simulink model "SchemaNL"  (R2020b)
settings: Solver=VariableStepAuto  StartTime=0.0  StopTime=50  RelTol=1e-3
values from neighbouring files (symbols this model uses):
  Kpsi = 0.5    [Coordinate_linearizzazione.m]
  Kx = 0.5    [Coordinate_linearizzazione.m]
  Ky = 0.5    [Coordinate_linearizzazione.m]
undefined symbols (not defined in the file or in its folder): DELTA
settings Model: Creator=teora  LastModifiedBy=teora

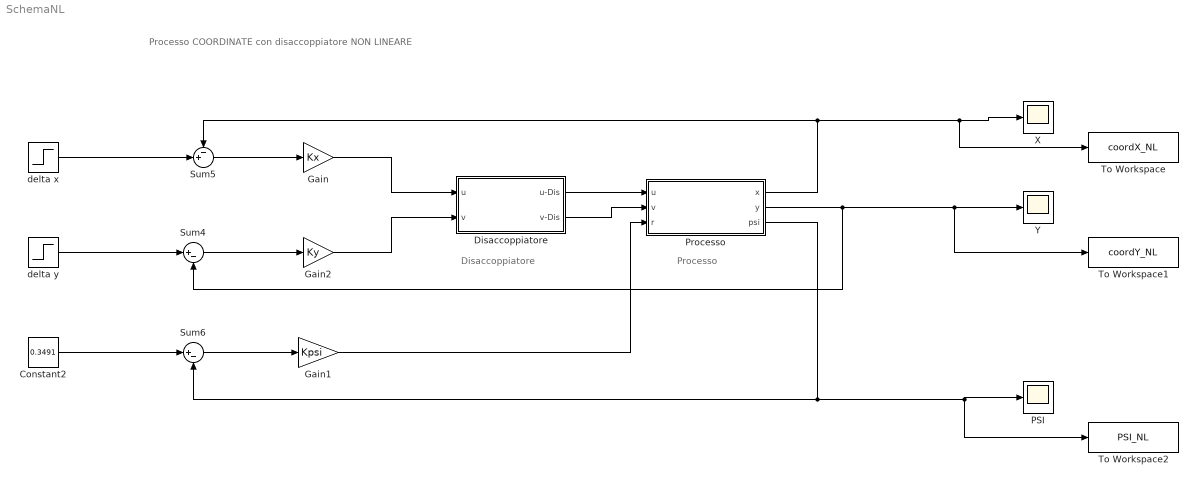
== system SchemaNL ==
  note: Processo
  note: Processo COORDINATE con disaccoppiatore NON LINEARE
  note: Disaccoppiatore
  Constant2 : Constant  Value=0.3491
  Disaccoppiatore : Subsystem
  Gain : Gain  Gain=Kx
  Gain1 : Gain  Gain=Kpsi
  Gain2 : Gain  Gain=Ky
  PSI : Scope
  Processo : Subsystem
  Sum4 : Sum  Inputs=|+-
  Sum5 : Sum  Inputs=-+|
  Sum6 : Sum  Inputs=|+-
  To Workspace : ToWorkspace  VariableName=coordX_NL  SaveFormat=Timeseries  SampleTime=-1
  To Workspace1 : ToWorkspace  VariableName=coordY_NL  SaveFormat=Timeseries  SampleTime=-1
  To Workspace2 : ToWorkspace  VariableName=PSI_NL  SaveFormat=Timeseries  SampleTime=-1
  X : Scope
  Y : Scope
  delta x : Step  Time=5  Before=5  After=10  SampleTime=0
  delta y : Step  Time=5  Before=10  After=10.5  SampleTime=0
  wires:
  Sum4/1 -> Gain2/1
  Sum5/1 -> Gain/1
  Constant2/1 -> Sum6/1
  Sum6/1 -> Gain1/1
  Gain/1 -> Disaccoppiatore/1(u)
  Gain2/1 -> Disaccoppiatore/2(v)
  delta x/1 -> Sum5/2
  delta y/1 -> Sum4/1
  Processo/2(y) -> Sum4/2, To Workspace1/1, Y/1
  Processo/1(x) -> X/1, To Workspace/1, Sum5/1
  Processo/3(psi) -> To Workspace2/1, PSI/1, Sum6/2
  Disaccoppiatore/1(u-Dis) -> Processo/1(u)
  Disaccoppiatore/2(v-Dis) -> Processo/2(v)
  Gain1/1 -> Processo/3(r)

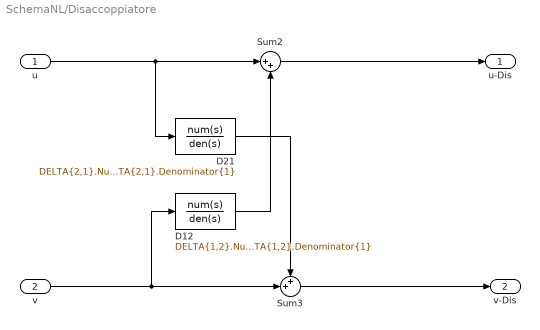
== system SchemaNL/Disaccoppiatore ==
  u : Inport
  v : Inport  Port=2
  D12 : TransferFcn  Numerator=DELTA{1,2}.Numerator{1}  Denominator=DELTA{1,2}.Denominator{1}
  D21 : TransferFcn  Numerator=DELTA{2,1}.Numerator{1}  Denominator=DELTA{2,1}.Denominator{1}
  Sum2 : Sum  Inputs=|++
  Sum3 : Sum  Inputs=++|
  u-Dis : Outport
  v-Dis : Outport  Port=2
  wires:
  Sum3/1 -> v-Dis/1
  v/1 -> Sum3/2, D12/1
  u/1 -> D21/1, Sum2/1
  Sum2/1 -> u-Dis/1
  D21/1 -> Sum3/1
  D12/1 -> Sum2/2

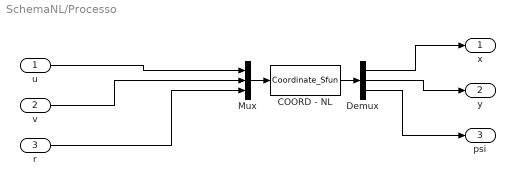
== system SchemaNL/Processo ==
  u : Inport
  v : Inport  Port=2
  r : Inport  Port=3
  COORD - NL : S-Function  FunctionName=Coordinate_Sfun  Parameters=x0  SFunctionDeploymentMode=off  EnableBusSupport=off
  Demux : Demux  Outputs=3
  Mux : Mux  Inputs=3
  x : Outport
  y : Outport  Port=2
  psi : Outport  Port=3
  wires:
  Mux/1 -> COORD - NL/1
  COORD - NL/1 -> Demux/1
  v/1 -> Mux/2
  Demux/2 -> y/1
  r/1 -> Mux/3
  Demux/1 -> x/1
  Demux/3 -> psi/1
  u/1 -> Mux/1
